simulink model "sampleModel1589"  (R2023a)
settings: Solver=VariableStepAuto  StartTime=0.0  StopTime=10.0  RelTol=1e-3
libraries: hdlsllib x3, simulink x2
settings Model: Creator=user1  LastModifiedBy=user1

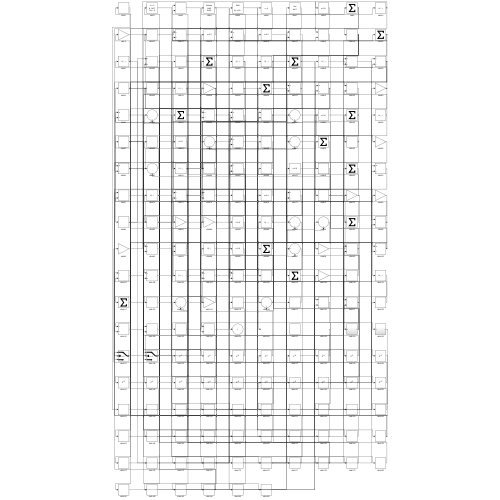
[thumbnail: Simulink's stored preview of the top-level diagram]
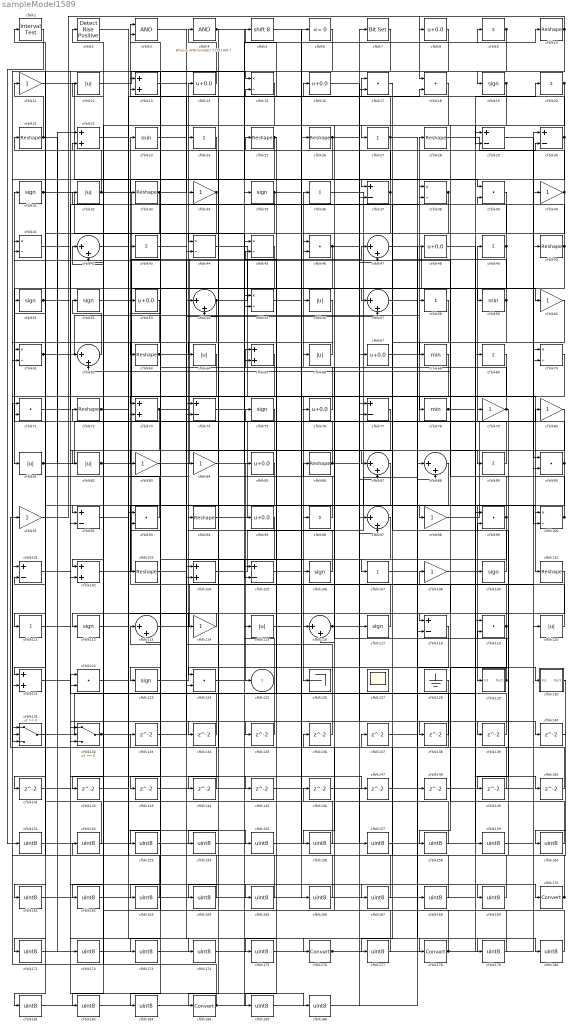
== system sampleModel1589 ==
  cfblk1 : hdlsllib/Logic and Bit Operations/Interval Test  IntervalClosedRight=on  uplimit=0.5  IntervalClosedLeft=on  lowlimit=-0.5  OutDataTypeStr=boolean
  cfblk{10,21,25..26,28,33,50,63,72,86,94,103,110} (13 alike) : Reshape
  cfblk{15,38,41,44..45,55,61,70,100} (9 alike) : Product  Inputs=*/  RndMeth=Zero  SaturateOnIntegerOverflow=on
  cfblk{29..30,37,74,77,92,101,105,118} (9 alike) : Sum  Inputs=+-
  cfblk{13,22,65,73,102,104,121} (7 alike) : Sum
  cfblk{19,31,35,51..52,75,106,109,112,117,123} (11 alike) : Signum
  cfblk{9,20,24,27,36,43,49,58,69,89,96,107,111} (13 alike) : Sum  Inputs=+
  cfblk{11,34,40,60,79..80,83..84,91,98,108,114} (12 alike) : Gain
  cfblk{42,47,54,57,62,87..88,97,113,116} (10 alike) : Sum  Inputs=|++
  cfblk{12,32,56,64,66,81..82,115,120} (9 alike) : Abs  SaturateOnIntegerOverflow=off
  cfblk{17..18,39,46,71,90,93,99,119,122,124} (11 alike) : DotProduct  OutDataTypeStr=Inherit: Inherit via internal rule
  cfblk126 : Terminator
  cfblk127 : Scope
      settings: Floating=on
  cfblk128 : Ground
  cfblk129 : Subsystem
      settings: LibrarySourceBlock=|
      | hdlsllib/Ports &
      | Subsystems/Subsystem
  cfblk130 : Subsystem
      settings: LibrarySourceBlock=|
      | hdlsllib/Ports &
      | Subsystems/Subsystem
  cfblk131 : Switch  SaturateOnIntegerOverflow=off  InputSameDT=off
  cfblk132 : Switch  SaturateOnIntegerOverflow=off  InputSameDT=off
  cfblk{133..150} (18 alike) : Delay  SampleTime=1
  cfblk{8,14,16,48,53,67,76,85,95} (9 alike) : Bias  Bias=0.0  SaturateOnIntegerOverflow=off
  cfblk{151..169,171..175,177,179..183,185..186} (32 alike) : DataTypeConversion  OutDataTypeStr=uint8  SaturateOnIntegerOverflow=off  RndMeth=Floor
  cfblk{170,176,178,184} (4 alike) : DataTypeConversion  SaturateOnIntegerOverflow=off  RndMeth=Floor
  cfblk2 : hdlsllib/Logic and Bit Operations/Detect Rise Positive  vinit=0  OutDataTypeStr=boolean
  cfblk{23,59,68,78} (4 alike) : MinMax
  cfblk3 : Logic  AllPortsSameDT=off  OutDataTypeStr=boolean
  cfblk4 : simulink/Logic and Bit Operations/Bitwise Operator  logicop=AND  UseBitMask=on  BitMask=bin2dec('11011001')  BitMaskRealWorld=Stored Integer
      settings: LibrarySourceBlock=|
      | hdlsllib/Logic and Bit
      | Operations/Bitwise
      | Operator
  cfblk5 : ArithShift  BitShiftNumber=8
  cfblk6 : hdlsllib/Logic and Bit Operations/Compare To Zero  relop=<=  OutDataTypeStr=boolean
  cfblk7 : simulink/Logic and Bit Operations/Bit Set  iBit=0
      settings: LibrarySourceBlock=|
      | hdlsllib/Logic and Bit
      | Operations/Bit Set
  cfblk125 : Outport  VectorParamsAs1DForOutWhenUnconnected=off
  wires:
  cfblk30/1 -> cfblk3/1, cfblk132/3, cfblk37/2, cfblk105/1
  cfblk97/1 -> cfblk184/1
  cfblk55/1 -> cfblk170/1
  cfblk90/1 -> cfblk28/1, cfblk171/1
  cfblk91/1 -> cfblk18/1
  cfblk36/1 -> cfblk129/1(In1)
  cfblk123/1 -> cfblk14/1
  cfblk79/1 -> cfblk36/1, cfblk149/1
  cfblk102/1 -> cfblk46/1
  cfblk86/1 -> cfblk31/1, cfblk47/2
  cfblk59/1 -> cfblk34/1, cfblk68/1
  cfblk99/1 -> cfblk41/1, cfblk105/2
  cfblk12/1 -> cfblk15/1
  cfblk56/1 -> cfblk102/1
  cfblk132/1 -> cfblk74/1, cfblk139/1
  cfblk4/1 -> cfblk44/1, cfblk39/1
  cfblk73/1 -> cfblk47/1, cfblk132/2, cfblk57/2
  cfblk119/1 -> cfblk23/1, cfblk158/1
  cfblk82/1 -> cfblk75/1, cfblk114/1
  cfblk70/1 -> cfblk73/1
  cfblk44/1 -> cfblk110/1
  cfblk50/1 -> cfblk39/2, cfblk143/1
  cfblk32/1 -> cfblk126/1, cfblk21/1
  cfblk98/1 -> cfblk80/1
  cfblk45/1 -> cfblk81/1
  cfblk128/1 -> cfblk91/1
  cfblk49/1 -> cfblk13/1, cfblk57/1
  cfblk37/1 -> cfblk22/2, cfblk182/1
  cfblk96/1 -> cfblk24/1
  cfblk35/1 -> cfblk44/2, cfblk167/1
  cfblk63/1 -> cfblk35/1, cfblk17/2
  cfblk66/1 -> cfblk63/1
  cfblk83/1 -> cfblk7/1
  cfblk47/1 -> cfblk60/1
  cfblk11/1 -> cfblk37/1
  cfblk61/1 -> cfblk56/1, cfblk172/1
  cfblk54/1 -> cfblk10/1, cfblk121/2
  cfblk93/1 -> cfblk51/1
  cfblk27/1 -> cfblk5/1, cfblk130/1(In1), cfblk121/1
  cfblk116/1 -> cfblk117/1, cfblk86/1
  cfblk38/1 -> cfblk64/1, cfblk164/1
  cfblk72/1 -> cfblk100/1, cfblk162/1
  cfblk34/1 -> cfblk141/1, cfblk142/1
  cfblk100/1 -> cfblk96/1, cfblk62/2
  cfblk42/1 -> cfblk178/1
  cfblk85/1 -> cfblk103/1
  cfblk58/1 -> cfblk87/1
  cfblk87/1 -> cfblk124/1
  cfblk113/1 -> cfblk40/1
  cfblk81/1 -> cfblk49/1, cfblk22/1
  cfblk84/1 -> cfblk125/1
  cfblk124/1 -> cfblk9/1
  cfblk33/1 -> cfblk92/1, cfblk17/1
  cfblk62/1 -> cfblk52/1
  cfblk25/1 -> cfblk183/1, cfblk185/1
  cfblk24/1 -> cfblk111/1
  cfblk15/1 -> cfblk33/1
  cfblk53/1 -> cfblk102/2
  cfblk64/1 -> cfblk131/2
  cfblk14/1 -> cfblk4/1
  cfblk3/1 -> cfblk106/1
  cfblk131/1 -> cfblk109/1
  cfblk52/1 -> cfblk59/1
  cfblk9/1 -> cfblk92/2, cfblk144/1
  cfblk67/1 -> cfblk38/1
  cfblk17/1 -> cfblk107/1
  cfblk129/1(Out1) -> cfblk94/1, cfblk66/1
  cfblk20/1 -> cfblk15/2, cfblk82/1
  cfblk48/1 -> cfblk119/1
  cfblk120/1 -> cfblk45/2
  cfblk112/1 -> cfblk84/1
  cfblk105/1 -> cfblk58/1
  cfblk114/1 -> cfblk112/1
  cfblk76/1 -> cfblk53/1
  cfblk46/1 -> cfblk87/2, cfblk175/1
  cfblk103/1 -> cfblk46/2
  cfblk117/1 -> cfblk3/2
  cfblk29/1 -> cfblk90/1
  cfblk40/1 -> cfblk122/2, cfblk25/1
  cfblk94/1 -> cfblk70/2
  cfblk10/1 -> cfblk19/1, cfblk8/1
  cfblk23/1 -> cfblk89/1
  cfblk60/1 -> cfblk98/1
  cfblk95/1 -> cfblk123/1
  cfblk111/1 -> cfblk132/1
  cfblk80/1 -> cfblk118/1
  cfblk21/1 -> cfblk11/1, cfblk62/1
  cfblk110/1 -> cfblk113/2
  cfblk122/1 -> cfblk18/2
  cfblk28/1 -> cfblk30/2
  cfblk89/1 -> cfblk12/1
  cfblk115/1 -> cfblk26/1
  cfblk106/1 -> cfblk65/1
  cfblk26/1 -> cfblk131/3, cfblk100/2
  cfblk8/1 -> cfblk61/1
  cfblk31/1 -> cfblk85/1, cfblk74/2
  cfblk71/1 -> cfblk38/2
  cfblk51/1 -> cfblk138/1, cfblk169/1, cfblk186/1
  cfblk7/1 -> cfblk61/2
  cfblk74/1 -> cfblk16/1
  cfblk19/1 -> cfblk29/2, cfblk116/1, cfblk78/1, cfblk124/2, cfblk116/2
  cfblk13/1 -> cfblk54/1
  cfblk65/1 -> cfblk104/2
  cfblk78/1 -> cfblk20/1, cfblk150/1
  cfblk109/1 -> cfblk41/2
  cfblk18/1 -> cfblk27/1
  cfblk43/1 -> cfblk176/1
  cfblk104/1 -> cfblk79/1
  cfblk75/1 -> cfblk83/1
  cfblk41/1 -> cfblk134/1
  cfblk134/1 -> cfblk73/2
  cfblk92/1 -> cfblk135/1
  cfblk135/1 -> cfblk45/1
  cfblk136/1 -> cfblk104/1
  cfblk138/1 -> cfblk65/2
  cfblk139/1 -> cfblk122/1
  cfblk16/1 -> cfblk140/1
  cfblk143/1 -> cfblk29/1
  cfblk144/1 -> cfblk113/1
  cfblk22/1 -> cfblk145/1
  cfblk145/1 -> cfblk118/2
  cfblk121/1 -> cfblk147/1
  cfblk147/1 -> cfblk70/1
  cfblk57/1 -> cfblk148/1
  cfblk148/1 -> cfblk30/1
  cfblk149/1 -> cfblk54/2
  cfblk150/1 -> cfblk13/2
  cfblk1/1 -> cfblk151/1
  cfblk151/1 -> cfblk120/1
  cfblk140/1 -> cfblk152/1
  cfblk152/1 -> cfblk1/1
  cfblk6/1 -> cfblk153/1
  cfblk153/1 -> cfblk76/1
  cfblk118/1 -> cfblk154/1
  cfblk154/1 -> cfblk6/1
  cfblk2/1 -> cfblk155/1
  cfblk155/1 -> cfblk67/1
  cfblk39/1 -> cfblk156/1
  cfblk156/1 -> cfblk2/1
  cfblk146/1 -> cfblk157/1
  cfblk157/1 -> cfblk90/2
  cfblk158/1 -> cfblk146/1
  cfblk108/1 -> cfblk159/1
  cfblk159/1 -> cfblk119/2
  cfblk130/1(Out1) -> cfblk160/1
  cfblk160/1 -> cfblk108/1
  cfblk69/1 -> cfblk161/1
  cfblk161/1 -> cfblk48/1
  cfblk162/1 -> cfblk69/1
  cfblk133/1 -> cfblk163/1
  cfblk163/1 -> cfblk71/2
  cfblk164/1 -> cfblk133/1
  cfblk101/1 -> cfblk165/1
  cfblk165/1 -> cfblk71/1
  cfblk5/1 -> cfblk166/1
  cfblk166/1 -> cfblk101/1
  cfblk167/1 -> cfblk101/2
  cfblk137/1 -> cfblk168/1
  cfblk168/1 -> cfblk93/1
  cfblk169/1 -> cfblk137/1
  cfblk170/1 -> cfblk99/2, cfblk72/1
  cfblk171/1 -> cfblk55/1
  cfblk172/1 -> cfblk55/2
  cfblk77/1 -> cfblk173/1
  cfblk173/1 -> cfblk95/1
  cfblk141/1 -> cfblk174/1
  cfblk174/1 -> cfblk77/1
  cfblk175/1 -> cfblk77/2
  cfblk176/1 -> cfblk99/1, cfblk50/1
  cfblk68/1 -> cfblk177/1
  cfblk177/1 -> cfblk43/1
  cfblk178/1 -> cfblk136/1, cfblk93/2
  cfblk107/1 -> cfblk179/1
  cfblk179/1 -> cfblk42/1
  cfblk142/1 -> cfblk180/1
  cfblk180/1 -> cfblk42/2
  cfblk88/1 -> cfblk181/1
  cfblk181/1 -> cfblk115/1
  cfblk182/1 -> cfblk88/1
  cfblk183/1 -> cfblk88/2
  cfblk184/1 -> cfblk32/1, cfblk131/1
  cfblk185/1 -> cfblk97/1
  cfblk186/1 -> cfblk97/2

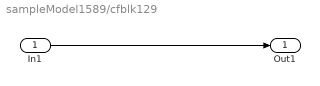
== system sampleModel1589/cfblk129 ==
  In1 : Inport
  Out1 : Outport
  wires:
  In1/1 -> Out1/1

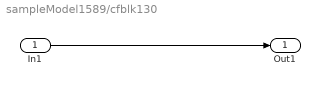
== system sampleModel1589/cfblk130 ==
  In1 : Inport
  Out1 : Outport
  wires:
  In1/1 -> Out1/1
